simulink model "pendolo"  (R2018b)
settings: Solver=VariableStepAuto  StartTime=0.0  StopTime=35  MaxStep=0.2  RelTol=1e-10
values from neighbouring files (symbols this model uses):
  g = 9.81    [pend.m]
  Jm = 3.1e-7    (= 3.1e-07)    [pend.m]
  Jp = 1774.274e-6    (= 0.001774274)    [pend.m]
  kd = 2    [pend.m]
  Kf = 7.44e-3    (= 0.00744)    [pend.m]
  kp = 20    [pend.m]
  La = 35e-6    (= 3.5e-05)    [pend.m]
  lb = 141.451e-3    (= 0.141451)    [pend.m]
  m = 135.4e-3    (= 0.1354)    [pend.m]
  M = 879.5e-3    (= 0.8795)    [pend.m]
  p1 = 0.0035    [cart_dumping.m]    (also in pend.m)
  p2 = 0.0058    [cart_dumping.m]    (also in pend.m)
  Ra = 3.92    [pend.m]
  Rg = 6.35e-3    (= 0.00635)    [pend.m]
  rt = 3.2067e-04    (= 0.00032067)    [pend.m]
  tet0 = pi/6    (= 0.523598775598)    [pend.m]
settings Model: Creator=lelli  LastModifiedBy=lelli
settings SFSimCC: SimUseLocalCustomCode=off
settings RTWCC: RTWUseLocalCustomCode=off

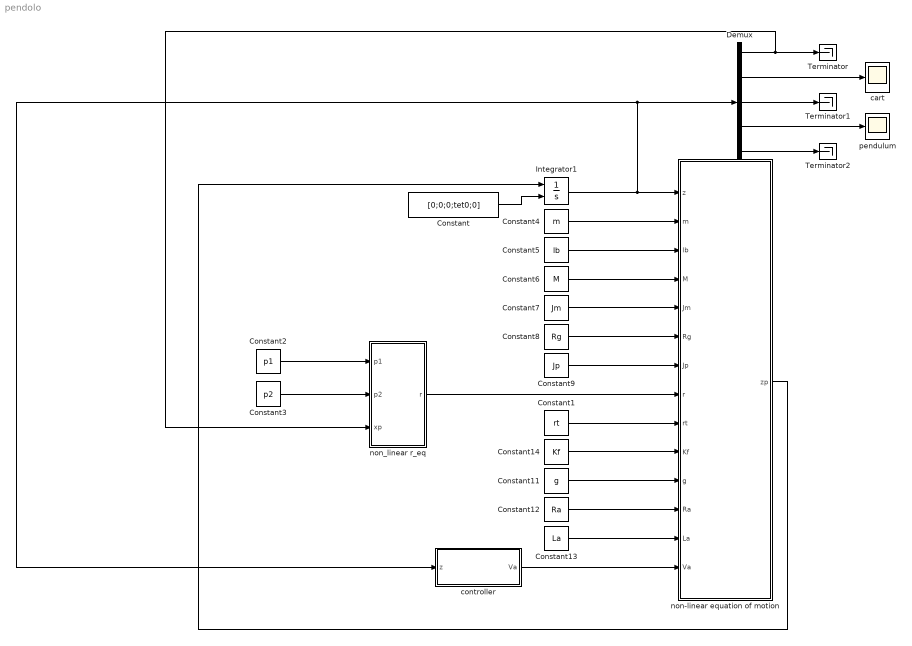
== system pendolo ==
  Constant : Constant  Value=[0;0;0;tet0;0]
  Constant1 : Constant  Value=rt
  Constant11 : Constant  Value=g
  Constant12 : Constant  Value=Ra
  Constant13 : Constant  Value=La
  Constant14 : Constant  Value=Kf
  Constant2 : Constant  Value=p1
  Constant3 : Constant  Value=p2
  Constant4 : Constant  Value=m
  Constant5 : Constant  Value=lb
  Constant6 : Constant  Value=M
  Constant7 : Constant  Value=Jm
  Constant8 : Constant  Value=Rg
  Constant9 : Constant  Value=Jp
  Demux : Demux  Outputs=5
  Integrator1 : Integrator  InitialConditionSource=external
  Terminator : Terminator
  Terminator1 : Terminator
  Terminator2 : Terminator
  cart : Scope
  controller : Subsystem
  "non-linear equation of motion " : MATLAB Function  TreatAsAtomicUnit=on
  "non_linear r_eq " : MATLAB Function  TreatAsAtomicUnit=on
  pendulum : Scope
  wires:
  Constant4/1 -> "non-linear equation of motion "/2(m)
  Constant5/1 -> "non-linear equation of motion "/3(lb)
  Constant6/1 -> "non-linear equation of motion "/4(M)
  Constant7/1 -> "non-linear equation of motion "/5(Jm)
  Constant8/1 -> "non-linear equation of motion "/6(Rg)
  Constant9/1 -> "non-linear equation of motion "/7(Jp)
  Constant14/1 -> "non-linear equation of motion "/10(Kf)
  Constant11/1 -> "non-linear equation of motion "/11(g)
  Constant12/1 -> "non-linear equation of motion "/12(Ra)
  Constant13/1 -> "non-linear equation of motion "/13(La)
  controller/1(Va) -> "non-linear equation of motion "/14(Va)
  Demux/2 -> cart/1
  Constant1/1 -> "non-linear equation of motion "/9(rt)
  "non_linear r_eq "/1(r) -> "non-linear equation of motion "/8(r)
  Constant2/1 -> "non_linear r_eq "/1(p1)
  Constant3/1 -> "non_linear r_eq "/2(p2)
  Constant/1 -> Integrator1/2
  Integrator1/1 -> Demux/1, controller/1(z), "non-linear equation of motion "/1(z)
  "non-linear equation of motion "/1(zp) -> Integrator1/1
  Demux/4 -> pendulum/1
  Demux/3 -> Terminator1/1
  Demux/5 -> Terminator2/1
  Demux/1 -> "non_linear r_eq "/3(xp), Terminator/1

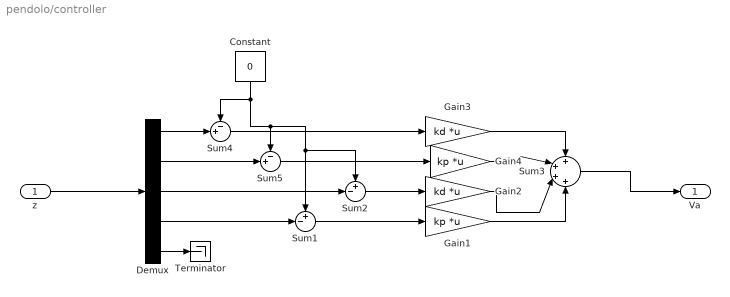
== system pendolo/controller ==
  z : Inport
  Constant : Constant  Value=0
  Demux : Demux  Outputs=5
  Gain1 : Gain  Gain=kp  Multiplication=Matrix(K*u)
  Gain2 : Gain  Gain=kd  Multiplication=Matrix(K*u)
  Gain3 : Gain  Gain=kd  Multiplication=Matrix(K*u)
  Gain4 : Gain  Gain=kp  Multiplication=Matrix(K*u)
  Sum1 : Sum  Inputs=+-|
  Sum2 : Sum  Inputs=+-|
  Sum3 : Sum  Inputs=++++
  Sum4 : Sum  Inputs=-+|
  Sum5 : Sum  Inputs=-+|
  Terminator : Terminator
  Va : Outport
  wires:
  Constant/1 -> Sum4/1, Sum2/1, Sum1/1, Sum5/1
  Demux/3 -> Sum2/2
  Gain2/1 -> Sum3/3
  Sum3/1 -> Va/1
  z/1 -> Demux/1
  Demux/4 -> Sum1/2
  Demux/1 -> Sum4/2
  Demux/2 -> Sum5/2
  Sum2/1 -> Gain2/1
  Sum1/1 -> Gain1/1
  Gain1/1 -> Sum3/4
  Demux/5 -> Terminator/1
  Sum5/1 -> Gain4/1
  Sum4/1 -> Gain3/1
  Gain4/1 -> Sum3/2
  Gain3/1 -> Sum3/1

== matlab function pendolo/non_linear r_eq  ==
  data: p1 input; r output; p2 input; xp input
function r  = r_eq(p1,p2,xp)
%non linear relationship between velocity and cart dumping
%p1 is the slope of linear approximation of force measured
%p2 is the intercept of linear approximation of force measured
%xp is the instantaneous velocity 
if xp>1e-16 || xp<-1e-16
    r=2*p2/pi*atan(100*xp)/xp + p1;
else
    r=2*p2/pi*100+p1;
end
end

== matlab function pendolo/non-linear equation of motion  ==
  data: z input; m input; zp output; lb input; M input; Jm input; Rg input; Jp input; r input; rt input; Kf input; g input; Ra input; La input; Va input
function zp = pendulum(z,m,lb,M,Jm,Rg,Jp,r,rt,Kf,g,Ra,La,Va)
xp=z(1);
tetap=z(3);
teta=z(4);
Ia=z(5);

A=[(M + m + Jm/Rg^2) 0 m*cos(teta)*lb 0 0; 
   0 1 0 0 0; 
   m*cos(teta)*lb 0 (Jp + m*lb^2) 0 0; 
   0 0 0 1 0; 
   0 0 0 0 La];

zp =(A)\[m*sin(teta)*lb*tetap^2 - r*xp - Kf*Ia/Rg;
         xp;
         - lb*m*g*sin(teta) - rt*tetap;
         tetap;
         Va - Ra*Ia + Kf/Rg*xp];
end
